simulink model "simulate"  (R2023a)
settings: Solver=VariableStepAuto  StartTime=0.0  StopTime=30  RelTol=1e-3
values from neighbouring files (symbols this model uses):
  KI = K(:,1:2)    [LQR_PI.m]    (also in full_loop.m = K(:,1:nref); inner_loop.m = K(:,1:3))
  Kp_x = K(:,3:5)    [LQR_PI.m]    (also in full_loop.m = K(:,nref+1:np+nref); inner_loop.m = K(:,4:9))
  Kp_xref = K(:,6:7)    [LQR_PI.m]    (also in full_loop.m = K(:,np+nref+1:end); inner_loop.m = K(:,10:12))
  sys_p = ss(Ap, Bp, Cp, Dp)    [LQR_PI.m]    (also in full_loop.m = ss(Ap, Bp, Cp([1:3,9],:), zeros(nref, mp)); inner_loop.m = ss(Ap(1:np, 1:np), Bp(1:np, :), Cp(:, 1:np), Dp))
  sys_ref = ss(A_ref, B_ref, C_ref, D_ref)    [LQR_PI.m]    (also in full_loop.m; inner_loop.m)
settings Model: Creator=timme  LastModifiedBy=timme

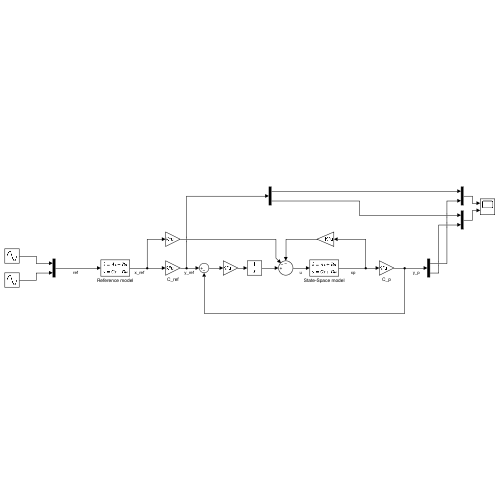
[thumbnail: Simulink's stored preview of the top-level diagram]
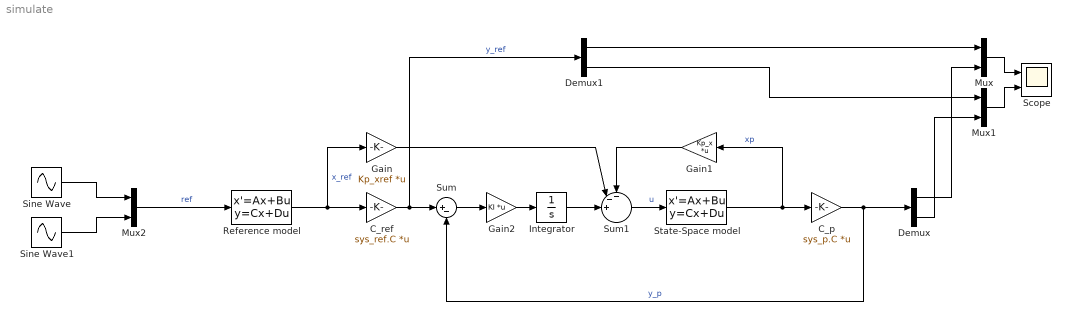
== system simulate ==
  C_p : Gain  Gain=sys_p.C  Multiplication=Matrix(K*u)
  C_ref : Gain  Gain=sys_ref.C  Multiplication=Matrix(K*u)
  Demux : Demux  Outputs=2
  Demux1 : Demux  Outputs=2
  Gain : Gain  Gain=Kp_xref  Multiplication=Matrix(K*u)
  Gain1 : Gain  Gain=Kp_x  Multiplication=Matrix(K*u)
  Gain2 : Gain  Gain=KI  Multiplication=Matrix(K*u)
  Integrator : Integrator
  Mux : Mux  Inputs=2
  Mux1 : Mux  Inputs=2
  Mux2 : Mux  Inputs=2
  Reference model : StateSpace  A=sys_ref.A  B=sys_ref.B  C=eye(2)  D=zeros(2,2)  InitialCondition=0
  Scope : Scope  NumInputPorts=2
  Sine Wave : Sin  Frequency=0.1  SampleTime=0
  Sine Wave1 : Sin  Frequency=0.3  SampleTime=0
  State-Space model : StateSpace  A=sys_p.A  B=sys_p.B  C=eye(3)  D=zeros(3,2)  InitialCondition=0
  Sum : Sum  Inputs=|+-
  Sum1 : Sum  Inputs=--+||
  wires:
  Reference model/1 -> C_ref/1, Gain/1  "x_ref"
  Mux2/1 -> Reference model/1  "ref"
  C_ref/1 -> Demux1/1, Sum/1  "y_ref"
  Sum/1 -> Gain2/1
  Gain/1 -> Sum1/2
  Sum1/1 -> State-Space model/1  "u"
  State-Space model/1 -> Gain1/1, C_p/1  "xp"
  C_p/1 -> Demux/1, Sum/2  "y_p"
  Gain1/1 -> Sum1/1
  Gain2/1 -> Integrator/1
  Demux/1 -> Mux/2
  Demux/2 -> Mux1/2
  Integrator/1 -> Sum1/3
  Demux1/1 -> Mux/1
  Demux1/2 -> Mux1/1
  Mux/1 -> Scope/1
  Mux1/1 -> Scope/2
  Sine Wave/1 -> Mux2/1
  Sine Wave1/1 -> Mux2/2
